simulink model "simu_control_ee1"  (R2021a)
settings: Solver=ode4  StartTime=0.0  StopTime=12  FixedStep=0.002  RelTol=1e-3
values from neighbouring files (symbols this model uses):
  A_d = eye(4)+A*T_s    [control_ee1.m]    (also in control_ee2.m; control_ee3.m)
  B_d = B*T_s    [control_ee1.m]    (also in control_ee2.m; control_ee3.m)
  F = inv(C_df*inv(eye(4)-(A_d+B_d*K))*B_d)    [control_ee2.m]
  K = place(A_d,-B_d,[exp(-T_s*15)+2e-4,exp(-T_s*5)+3e-4, exp(-T_s*15)+4e-4, exp(-T_s*8)])    [control_ee1.m]    (also in control_ee2.m; control_ee3.m)
  KH = acker(A_dext, -B_dext, [exp(-T_s*10)+2e-4,exp(-T_s*3)+3e-4, exp(-T_s*10)+4e-4, exp(-T_s*8), exp(-T_s*10)])    [control_ee3.m]
  L = L'    [control_ee1.m]    (also in control_ee2.m; control_ee3.m)
undefined symbols (not defined in the file or in its folder): DiscIntNeverNeededParam
libraries: simulink x3
settings Model: Creator=frand  LastModifiedBy=frand

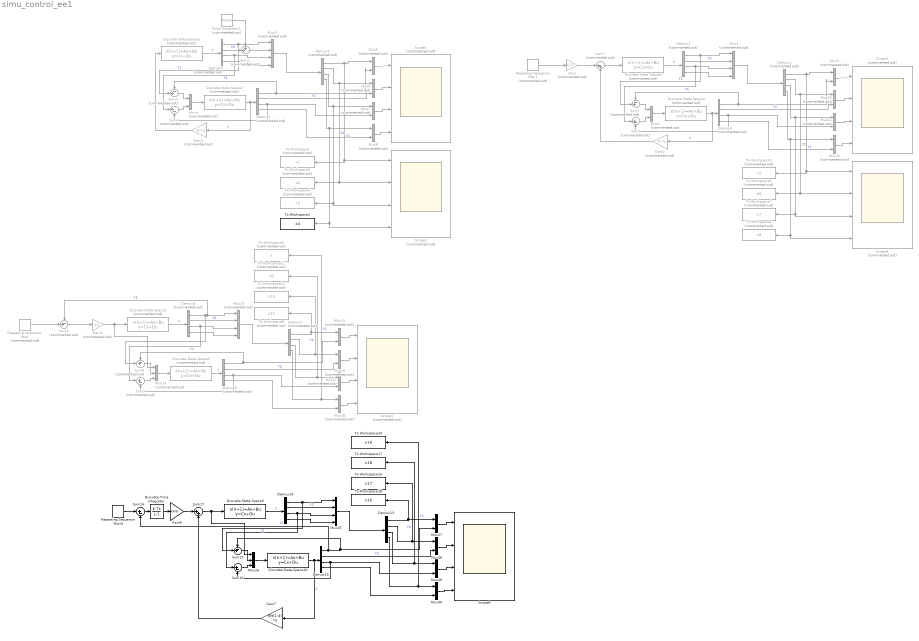
== system simu_control_ee1 ==
  Demux{1..9} (9 alike) : Demux  Commented=on
  Demux13 : Demux
  Demux14 : Demux
  Demux15 : Demux
  Discrete State-Space1 : DiscreteStateSpace  Commented=on  A=A_d  B=B_d  C=eye(4)  D=[0;0;0;0]  InitialCondition=[-12.92;0;0;0]  SampleTime=0.02
  Discrete State-Space10 : DiscreteStateSpace  A=A_d  B=[B_d,L]  C=eye(4)  D=0*[B_d,L]  InitialCondition=[0;0;0;0]  SampleTime=0.02
  Discrete State-Space2 : DiscreteStateSpace  Commented=on  A=A_d+B_d*K  B=L  C=eye(4)  D=0*L  InitialCondition=[0;0;0;0]  SampleTime=0.02
  Discrete State-Space3 : DiscreteStateSpace  Commented=on  A=A_d  B=B_d  C=eye(4)  D=[0;0;0;0]  InitialCondition=[0;0;0;0]  SampleTime=0.02
  Discrete State-Space4 : DiscreteStateSpace  Commented=on  A=A_d+B_d*K  B=L  C=eye(4)  D=0*L  InitialCondition=[0;0;0;0]  SampleTime=0.02
  Discrete State-Space5 : DiscreteStateSpace  Commented=on  A=A_d  B=B_d  C=eye(4)  D=[0;0;0;0]  InitialCondition=[0;0;0;0]  SampleTime=0.02
  Discrete State-Space6 : DiscreteStateSpace  Commented=on  A=A_d  B=[B_d,L]  C=eye(4)  D=0*[B_d,L]  InitialCondition=[0;0;0;0]  SampleTime=0.02
  Discrete State-Space9 : DiscreteStateSpace  A=A_d  B=B_d  C=eye(4)  D=[0;0;0;0]  InitialCondition=[0;0;0;0]  SampleTime=0.02
  Discrete-Time Integrator : DiscreteIntegrator  SampleTime=-1  ICPrevOutput=DiscIntNeverNeededParam  ICPrevScaledInput=DiscIntNeverNeededParam
  Gain : Gain  Commented=on  Gain=F(1)
  Gain1 : Gain  Commented=on  Gain=K  Multiplication=Matrix(K*u)
  Gain2 : Gain  Commented=on  Gain=K  Multiplication=Matrix(K*u)
  Gain3 : Gain  Commented=on  Gain=-1.5
  Gain6 : Gain  Gain=KH(5)
  Gain7 : Gain  Gain=KH(1:4)  Multiplication=Matrix(K*u)
  Mux1 : Mux  Commented=on
  Mux{2,4..12,15..18} (14 alike) : Mux  Commented=on  Inputs=2
  Mux13 : Mux  Commented=on
  Mux14 : Mux  Commented=on  Inputs=3
  Mux25 : Mux
  Mux26 : Mux  Inputs=3
  Mux{27..30} (4 alike) : Mux  Inputs=2
  Mux3 : Mux  Commented=on
  Pulse Generator1 : DiscretePulseGenerator  Commented=on  PulseType=Time based  Amplitude=-151*0  Period=50  PulseWidth=0.02*10  PhaseDelay=1
  Repeating Sequence Stair : simulink/Sources/Repeating Sequence Stair  Commented=on  OutValues=[-8 0 8 0].'  tsamp=2.4  OutMin=[]  OutMax=[]  OutDataTypeStr=double  OutputDataTypeScalingMode=double  OutDataType=fixdt(0,8)  ConRadixGroup=Best Precision: Vector-wise  OutScaling=2^-12
  Repeating Sequence Stair1 : simulink/Sources/Repeating Sequence Stair  Commented=on  OutValues=[10 0 -10 0].'  tsamp=3  OutMin=[]  OutMax=[]  OutDataTypeStr=double  OutputDataTypeScalingMode=double  OutDataType=fixdt(0,8)  ConRadixGroup=Best Precision: Vector-wise  OutScaling=2^-12
  Repeating Sequence Stair3 : simulink/Sources/Repeating Sequence Stair  OutValues=[10 0 -10 0].'  tsamp=3  OutMin=[]  OutMax=[]  OutDataTypeStr=double  OutputDataTypeScalingMode=double  OutDataType=fixdt(0,8)  ConRadixGroup=Best Precision: Vector-wise  OutScaling=2^-12
  Scope{1..5} (5 alike) : Scope  Commented=on  NumInputPorts=4
  Scope8 : Scope  NumInputPorts=4
  Sum{1,3,5,8} (4 alike) : Sum  Commented=on  Inputs=-+|
  Sum14 : Sum  Inputs=|+-
  Sum15 : Sum  Inputs=-+|
  Sum16 : Sum  Inputs=|+-
  Sum17 : Sum  Inputs=|++
  Sum2 : Sum  Commented=on  Inputs=++|
  Sum4 : Sum  Commented=on  Inputs=|+-
  Sum6 : Sum  Commented=on  Inputs=|+-
  Sum7 : Sum  Commented=on  Inputs=|++
  Sum9 : Sum  Commented=on  Inputs=|+-
  To Workspace : ToWorkspace  Commented=on  VariableName=x1  SampleTime=-1
  To Workspace1 : ToWorkspace  VariableName=x4  SampleTime=-1
  To Workspace10 : ToWorkspace  Commented=on  VariableName=x10  SampleTime=-1
  To Workspace11 : ToWorkspace  Commented=on  VariableName=x9  SampleTime=-1
  To Workspace16 : ToWorkspace  VariableName=x17  SampleTime=-1
  To Workspace17 : ToWorkspace  VariableName=x18  SampleTime=-1
  To Workspace18 : ToWorkspace  VariableName=x16  SampleTime=-1
  To Workspace19 : ToWorkspace  VariableName=x19  SampleTime=-1
  To Workspace2 : ToWorkspace  Commented=on  VariableName=x2  SampleTime=-1
  To Workspace3 : ToWorkspace  Commented=on  VariableName=x3  SampleTime=-1
  To Workspace4 : ToWorkspace  Commented=on  VariableName=x8  SampleTime=-1
  To Workspace5 : ToWorkspace  Commented=on  VariableName=x5  SampleTime=-1
  To Workspace6 : ToWorkspace  Commented=on  VariableName=x6  SampleTime=-1
  To Workspace7 : ToWorkspace  Commented=on  VariableName=x7  SampleTime=-1
  To Workspace8 : ToWorkspace  Commented=on  VariableName=x11  SampleTime=-1
  To Workspace9 : ToWorkspace  Commented=on  VariableName=x  SampleTime=-1
  wires:
  Gain1/1 -> Discrete State-Space1/1
  Discrete State-Space1/1 -> Demux4/1  "Y"
  Mux3/1 -> Demux3/1
  Demux4/4 -> Mux3/4
  Demux4/3 -> Sum4/1, Mux3/3
  Pulse Generator1/1 -> Sum2/1
  Demux3/1 -> To Workspace/1, Scope2/1, Mux5/1  "Y1"
  Mux5/1 -> Scope1/1
  Demux5/1 -> Mux5/2, Sum3/1  "Y1"
  Demux3/2 -> To Workspace2/1, Scope2/2, Mux6/1  "Y2"
  Demux5/2 -> Mux6/2  "Y2"
  Demux3/3 -> To Workspace3/1, Scope2/3, Mux7/1
  Demux3/4 -> Scope2/4, To Workspace1/1, Mux8/1
  Demux5/3 -> Mux7/2, Sum4/2
  Demux5/4 -> Mux8/2
  Mux6/1 -> Scope1/2
  Mux7/1 -> Scope1/3
  Mux8/1 -> Scope1/4
  Discrete State-Space2/1 -> Gain1/1, Demux5/1  "Y"
  Mux4/1 -> Discrete State-Space2/1
  Sum4/1 -> Mux4/2
  Sum3/1 -> Mux4/1
  Demux4/2 -> Sum2/2  "Y2"
  Sum2/1 -> Mux3/2
  Demux4/1 -> Sum3/2, Mux3/1  "Y1"
  Sum6/1 -> Mux2/2
  Sum5/1 -> Mux2/1
  Mux10/1 -> Scope3/2
  Demux6/4 -> Mux12/2
  Demux1/3 -> To Workspace7/1, Scope4/3, Mux11/1
  Mux2/1 -> Discrete State-Space4/1
  Mux9/1 -> Scope3/1
  Demux1/2 -> To Workspace6/1, Scope4/2, Mux10/1  "Y2"
  Mux12/1 -> Scope3/4
  Demux1/1 -> To Workspace5/1, Scope4/1, Mux9/1  "Y1"
  Demux6/3 -> Mux11/2, Sum6/2
  Mux11/1 -> Scope3/3
  Discrete State-Space3/1 -> Demux2/1  "Y"
  Demux1/4 -> Scope4/4, To Workspace4/1, Mux12/1
  Demux6/2 -> Mux10/2  "Y2"
  Demux6/1 -> Mux9/2, Sum5/1  "Y1"
  Demux2/1 -> Sum5/2, Mux1/1  "Y1"
  Mux1/1 -> Demux1/1
  Demux2/2 -> Mux1/2  "Y2"
  Demux2/3 -> Sum6/1, Mux1/3
  Demux2/4 -> Mux1/4
  Discrete State-Space4/1 -> Gain2/1, Demux6/1  "Y"
  Gain/1 -> Sum7/1
  Sum7/1 -> Discrete State-Space3/1
  Gain2/1 -> Sum7/2
  Demux8/1 -> Sum1/1, Mux13/1, Sum8/2  "Y1"
  Demux8/2 -> Mux13/2  "Y2"
  Sum8/1 -> Mux14/2
  Sum9/1 -> Mux14/3
  Mux14/1 -> Discrete State-Space6/1
  Discrete State-Space6/1 -> Demux9/1  "Y"
  Mux18/1 -> Scope5/4
  Mux17/1 -> Scope5/3
  Mux16/1 -> Scope5/2
  Demux9/4 -> Mux18/2
  Demux9/3 -> Sum9/2, Mux17/2
  Demux7/4 -> Mux18/1, To Workspace9/1
  Demux7/3 -> Mux17/1, To Workspace11/1
  Demux9/2 -> Mux16/2  "Y2"
  Demux7/2 -> To Workspace10/1, Mux16/1  "Y2"
  Demux9/1 -> Sum8/1, Mux15/2  "Y1"
  Mux15/1 -> Scope5/1
  Demux7/1 -> To Workspace8/1, Mux15/1  "Y1"
  Demux8/3 -> Mux13/3, Sum9/1
  Demux8/4 -> Mux13/4
  Mux13/1 -> Demux7/1
  Discrete State-Space5/1 -> Demux8/1  "Y"
  Sum1/1 -> Gain3/1
  Gain3/1 -> Mux14/1, Discrete State-Space5/1
  Repeating Sequence Stair/1 -> Sum1/2
  Repeating Sequence Stair1/1 -> Gain/1
  Repeating Sequence Stair3/1 -> Sum14/1
  Sum14/1 -> Discrete-Time Integrator/1
  Discrete State-Space9/1 -> Demux14/1  "Y"
  Mux25/1 -> Demux13/1
  Demux14/4 -> Mux25/4
  Demux14/3 -> Sum16/1, Mux25/3
  Demux13/1 -> Mux27/1, To Workspace18/1  "Y1"
  Mux27/1 -> Scope8/1
  Demux15/1 -> Mux27/2, Sum15/1, Sum14/2  "Y1"
  Demux13/2 -> Mux28/1, To Workspace16/1  "Y2"
  Demux15/2 -> Mux28/2  "Y2"
  Demux13/3 -> To Workspace17/1, Mux29/1
  Demux13/4 -> To Workspace19/1, Mux30/1
  Demux15/3 -> Mux29/2, Sum16/2
  Demux15/4 -> Mux30/2
  Mux28/1 -> Scope8/2
  Mux29/1 -> Scope8/3
  Mux30/1 -> Scope8/4
  Discrete State-Space10/1 -> Gain7/1, Demux15/1  "Y"
  Mux26/1 -> Discrete State-Space10/1
  Sum16/1 -> Mux26/3
  Sum15/1 -> Mux26/2
  Demux14/2 -> Mux25/2  "Y2"
  Demux14/1 -> Mux25/1, Sum15/2  "Y1"
  Gain7/1 -> Sum17/2
  Gain6/1 -> Sum17/1
  Sum17/1 -> Mux26/1, Discrete State-Space9/1
  Discrete-Time Integrator/1 -> Gain6/1
